simulink model "astolfi_278334"  (R2024b)
settings: Solver=ode113  StartTime=0.0  StopTime=60  RelTol=1e-10
values from neighbouring files (symbols this model uses):
  Ic = Iz + 2*Izz + 2*Mk*L*L    (= 7.5230625)    [Astolfi_278334.m]    (also in astolfi_278334.m)
  Ixx = (1/2)*Mk*Rk*Rk    (= 0.0140625)    [Astolfi_278334.m]    (also in astolfi_278334.m)
  k1 = 1    [Astolfi_278334.m]    (also in astolfi_278334.m)
  k2 = 10    [Astolfi_278334.m]    (also in astolfi_278334.m)
  Kd = 10    [Astolfi_278334.m]    (also in astolfi_278334.m)
  L = 0.3    [Astolfi_278334.m]    (also in astolfi_278334.m)
  Mc = Mp + 2*Mk    (= 107)    [Astolfi_278334.m]    (also in astolfi_278334.m)
  q0 = [1; 1;   pi;    0;    0]    [Astolfi_278334.m]    (also in astolfi_278334.m = [0; 0;   0;    0;    0])
  Rk = 0.075    [Astolfi_278334.m]    (also in astolfi_278334.m)
  thetad0 = 0    [Astolfi_278334.m]    (also in astolfi_278334.m)
  vd = wd*Rd    (= 1.0471975512)    [Astolfi_278334.m]    (also in astolfi_278334.m)
  wd = pi/6    (= 0.523598775598)    [Astolfi_278334.m]    (also in astolfi_278334.m)
  xd0 = 5    [Astolfi_278334.m]    (also in astolfi_278334.m)
  yd0 = -3    [Astolfi_278334.m]    (also in astolfi_278334.m)
settings Model: Creator=radek  LastModifiedBy=radek

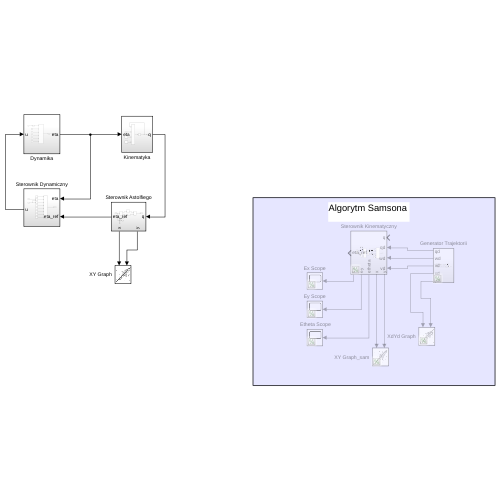
[thumbnail: Simulink's stored preview of the top-level diagram]
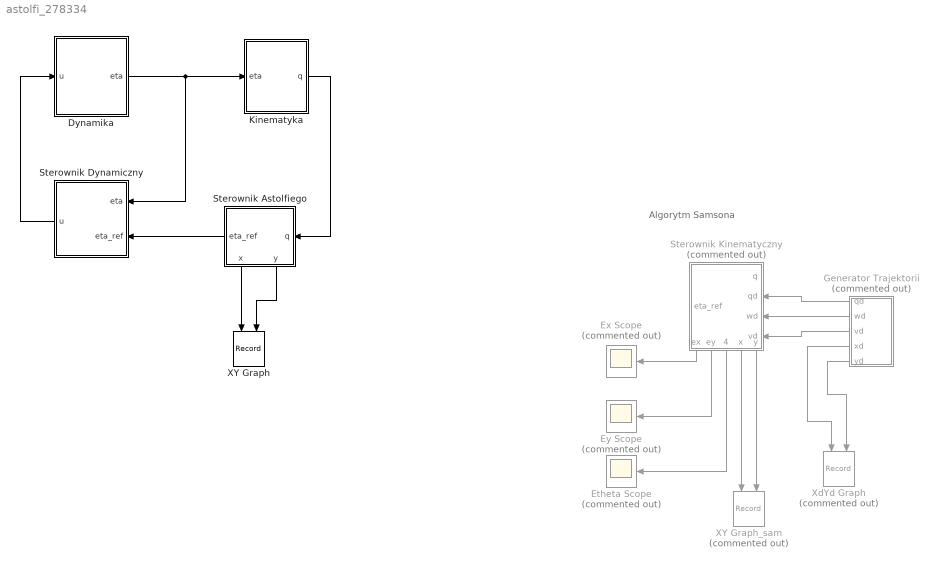
== system astolfi_278334 ==
  note: Algorytm Samsona
  " Etheta Scope" : Scope  Commented=on
  Dynamika : Subsystem
  Ex Scope : Scope  Commented=on
  Ey Scope : Scope  Commented=on
  Generator Trajektorii : Subsystem  Commented=on
  Kinematyka : Subsystem
  Sterownik Astolfiego : Subsystem
      settings: PortSchema="{\"entries\":[{\"content\":{\"sides\":[{\"content\":{\"connectorIds\":[\"In1\"]},\"type\":\"ConnectorPlacement.EquallySpacedRectSide\",\"uuid\":\"f5e69acf-f3ff-4fdf-98d6-c8734f1034ce\"},{\"content\":{\"connectorIds\":[\"Out1\"],\"side\":\"RIGHT\"},\"type\":\"ConnectorPlacement.EquallySpacedRectSide\",\"uuid\":\"aebf7805-5044-4096-9d39-e64456f3e00a\"},{\"content\":{\"side\":\"TOP\"},\"type\":\"ConnectorPlacement.EquallySpacedRectSide\",\"uuid\":\"74c1e2cd-73e2-4d01-a630-37efeb3275a2\"},{\"content\":{\"connectorIds\":[\"Out2\",\"Out3\"],\"side\":\"BOTTOM\"},\"type\":\"ConnectorPlacement.EquallySpacedRectSide\",\"uuid\":\"5cf9958d-65eb-4d7e-96d9-423271126dc6\"}]},\"type\":\"ConnectorPlacement.EquallySpacedConnector\",\"uuid\":\"6917b8e7-ecbe-45a3-8115-cac047f2c7ac\"}],\"packageUris\":[\"http://schema.mathworks.com/mf0/Connector/R2020b\"],\"version\":\"1.0\"}"
  Sterownik Dynamiczny : Subsystem
  Sterownik Kinematyczny : Subsystem  Commented=on
      settings: PortSchema="{\"entries\":[{\"content\":{\"sides\":[{\"content\":{\"connectorIds\":[\"In1\",\"In2\",\"In3\",\"In4\"]},\"type\":\"ConnectorPlacement.EquallySpacedRectSide\",\"uuid\":\"5192a1cc-ed77-4e56-a122-cfee3012277d\"},{\"content\":{\"connectorIds\":[\"Out1\"],\"side\":\"RIGHT\"},\"type\":\"ConnectorPlacement.EquallySpacedRectSide\",\"uuid\":\"40a037b4-09b0-4e17-a01c-e9007902fa24\"},{\"content\":{\"side\":\"TOP\"},\"type\":\"ConnectorPlacement.EquallySpacedRectSide\",\"uuid\":\"cd491b5b-2c4b-4e8a-9ff0-8dca4b136ad7\"},{\"content\":{\"connectorIds\":[\"Out2\",\"Out3\",\"Out4\",\"Out5\",\"Out6\"],\"side\":\"BOTTOM\"},\"type\":\"ConnectorPlacement.EquallySpacedRectSide\",\"uuid\":\"bb7d56d9-1ae6-4c8e-b63d-595b22e12c82\"}]},\"type\":\"ConnectorPlacement.EquallySpacedConnector\",\"uuid\":\"47c22155-c6cc-44ec-a96c-4ab3b3072b69\"}],\"packageUris\":[\"http://schema.mathworks.com/mf0/Connector/R2020b\"],\"version\":\"1.0\"}"
  XY Graph : Record  FileSettingsInternal="{\"entries\":[{\"content\":{\"excelSettings\":{\"content\":{},\"type\":\"Streamout.ExcelSettings\"}},\"type\":\"Streamout.FileSettingStorage\",\"uuid\":\"\"}],\"packageUris\":[\"http:\\/\\/schema.mathworks.com\\/mf0\\/streamout_blocks\\/R2020a\"],\"version\":\"1.0\"}"  Layout=[1 1]  SignalsInternal="{\"entries\":[{\"content\":{\"signals\":[{\"content\":{\"blockPath\":[],\"dimensions\":[1,1],\"domain\":\"\",\"lineColor\":\"#0072bd\",\"plots\":[ 1 ],\"port\":1,\"sid\":[\"\"],\"signalID\":1,\"signalName\":\"Sterownik Astolfiego:3\"},\"type\":\"RecordBlkView.Signal\",\"uuid\":\"\"},{\"content\":{\"blockPath\":[],\"dimensions\":[1,1],\"domain\":\"\",\"lineColor\":\"#d95319\",\"plots\":[ 1 ],\"port\":2,\"sid\":[\"\"],\"signalID\":2,\"signalName\":\"Sterownik Astolfiego:2\"},\"type\":\"RecordBlkView.Signal\",\"uuid\":\"\"}]},\"type\":\"RecordBlkView.InputSignals\",\"uuid\":\"\"}],\"packageUris\":[\"http:\\/\\/schema.mathworks.com\\/mf0\\/streamout_blocks\\/R2020a\"],\"version\":\"1.0\"}"  VisualizationBindings="{\"xyplotplugin\":{\"info\":[{\"series\":[{\"bindingParametersList\":[{\"parameter\":\"X-Axis\",\"signalID\":1,\"signalName\":\"Sterownik Astolfiego:3\"},{\"parameter\":\"Y-Axis\",\"signalID\":2,\"signalName\":\"Sterownik Astolfiego:2\"}],\"seriesID\":0}],\"subplotID\":1}]}}"  CompatibilityTag=XY
  XY Graph_sam : Record  Commented=on  FileSettingsInternal="{\"entries\":[{\"content\":{\"excelSettings\":{\"content\":{},\"type\":\"Streamout.ExcelSettings\"}},\"type\":\"Streamout.FileSettingStorage\",\"uuid\":\"\"}],\"packageUris\":[\"http:\\/\\/schema.mathworks.com\\/mf0\\/streamout_blocks\\/R2020a\"],\"version\":\"1.0\"}"  Layout=[1 1]  SignalsInternal="{\"entries\":[{\"content\":{\"signals\":[{\"content\":{\"blockPath\":[],\"dimensions\":[1],\"domain\":\"\",\"lineColor\":\"#0072bd\",\"plots\":[ 1 ],\"port\":1,\"signalID\":1,\"signalName\":\"Sterownik Kinematyczny:3\"},\"type\":\"RecordBlkView.Signal\",\"uuid\":\"\"},{\"content\":{\"blockPath\":[],\"dimensions\":[1],\"domain\":\"\",\"lineColor\":\"#d95319\",\"plots\":[ 1 ],\"port\":2,\"signalID\":2,\"signalName\":\"Sterownik Kinematyczny:2\"},\"type\":\"RecordBlkView.Signal\",\"uuid\":\"\"}]},\"type\":\"RecordBlkView.InputSignals\",\"uuid\":\"\"}],\"packageUris\":[\"http:\\/\\/schema.mathworks.com\\/mf0\\/streamout_blocks\\/R2020a\"],\"version\":\"1.0\"}"  VisualizationBindings="{\"xyplotplugin\":{\"info\":[{\"series\":[{\"bindingParametersList\":[{\"parameter\":\"X-Axis\",\"signalID\":1,\"signalName\":\"Sterownik Kinematyczny:3\"},{\"parameter\":\"Y-Axis\",\"signalID\":2,\"signalName\":\"Sterownik Kinematyczny:2\"}],\"seriesID\":0}],\"subplotID\":1}]}}"  CompatibilityTag=XY
  XdYd Graph : Record  Commented=on  FileSettingsInternal="{\"entries\":[{\"content\":{\"excelSettings\":{\"content\":{},\"type\":\"Streamout.ExcelSettings\"}},\"type\":\"Streamout.FileSettingStorage\",\"uuid\":\"\"}],\"packageUris\":[\"http:\\/\\/schema.mathworks.com\\/mf0\\/streamout_blocks\\/R2020a\"],\"version\":\"1.0\"}"  Layout=[1 1]  SignalsInternal="{\"entries\":[{\"content\":{\"signals\":[{\"content\":{\"blockPath\":[],\"dimensions\":[1],\"domain\":\"\",\"lineColor\":\"#a2142f\",\"plots\":[ 1 ],\"port\":1,\"signalID\":1,\"signalName\":\"Generator Trajektorii:4\"},\"type\":\"RecordBlkView.Signal\",\"uuid\":\"\"},{\"content\":{\"blockPath\":[],\"dimensions\":[1],\"domain\":\"\",\"lineColor\":\"#139fff\",\"plots\":[ 1 ],\"port\":2,\"signalID\":2,\"signalName\":\"Generator Trajektorii:5\"},\"type\":\"RecordBlkView.Signal\",\"uuid\":\"\"}]},\"type\":\"RecordBlkView.InputSignals\",\"uuid\":\"\"}],\"packageUris\":[\"http:\\/\\/schema.mathworks.com\\/mf0\\/streamout_blocks\\/R2020a\"],\"version\":\"1.0\"}"  VisualizationBindings="{\"xyplotplugin\":{\"info\":[{\"series\":[{\"bindingParametersList\":[{\"parameter\":\"X-Axis\",\"signalID\":1,\"signalName\":\"Generator Trajektorii:4\"},{\"parameter\":\"Y-Axis\",\"signalID\":2,\"signalName\":\"Generator Trajektorii:5\"}],\"seriesID\":0}],\"subplotID\":1}]}}"  CompatibilityTag=XY
  wires:
  Dynamika/1(eta) -> Sterownik Dynamiczny/1(eta), Kinematyka/1(eta)
  Sterownik Dynamiczny/1(u) -> Dynamika/1(u)
  Generator Trajektorii/1(qd) -> Sterownik Kinematyczny/2(qd)
  Generator Trajektorii/2(wd) -> Sterownik Kinematyczny/3(wd)
  Generator Trajektorii/3(vd) -> Sterownik Kinematyczny/4(vd)
  Sterownik Kinematyczny/3(x) -> XY Graph_sam/1
  Sterownik Kinematyczny/2(y) -> XY Graph_sam/2
  Generator Trajektorii/4(xd) -> XdYd Graph/1
  Generator Trajektorii/5(yd) -> XdYd Graph/2
  Sterownik Kinematyczny/6(ex) -> Ex Scope/1
  Sterownik Kinematyczny/5(ey) -> Ey Scope/1
  Sterownik Kinematyczny/4(etheta) -> " Etheta Scope"/1
  Sterownik Astolfiego/1(eta_ref) -> Sterownik Dynamiczny/2(eta_ref)
  Kinematyka/1(q) -> Sterownik Astolfiego/1(q)
  Sterownik Astolfiego/3(x) -> XY Graph/1
  Sterownik Astolfiego/2(y) -> XY Graph/2

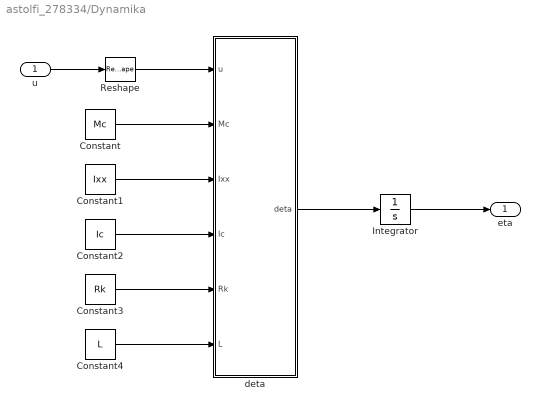
== system astolfi_278334/Dynamika ==
  u : Inport
  Constant : Constant  Value=Mc
  Constant1 : Constant  Value=Ixx
  Constant2 : Constant  Value=Ic
  Constant3 : Constant  Value=Rk
  Constant4 : Constant  Value=L
  Integrator : Integrator
  Reshape : Reshape  OutputDimensionality=Customize  OutputDimensions=[2,1]
  deta : MATLAB Function  TreatAsAtomicUnit=on
  eta : Outport
  wires:
  u/1 -> Reshape/1
  Constant1/1 -> deta/3(Ixx)
  Constant3/1 -> deta/5(Rk)
  Constant2/1 -> deta/4(Ic)
  Constant/1 -> deta/2(Mc)
  Constant4/1 -> deta/6(L)
  Integrator/1 -> eta/1
  deta/1(deta) -> Integrator/1
  Reshape/1 -> deta/1(u)

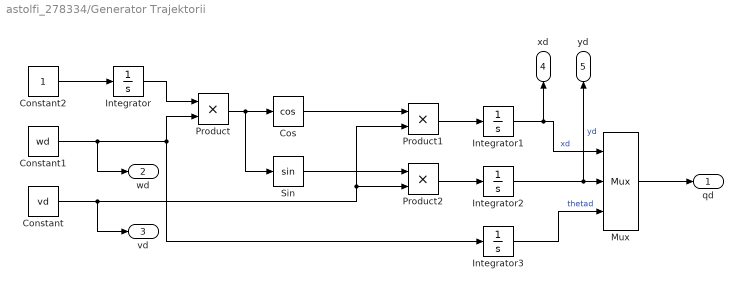
== system astolfi_278334/Generator Trajektorii ==
  Constant : Constant  Value=vd
  Constant1 : Constant  Value=wd
  Constant2 : Constant
  Cos : Trigonometry  Operator=cos
  Integrator : Integrator
  Integrator1 : Integrator  InitialCondition=xd0
  Integrator2 : Integrator  InitialCondition=yd0
  Integrator3 : Integrator  InitialCondition=thetad0
  Mux : Mux  Inputs=3
  Product : Product
  Product1 : Product
  Product2 : Product
  Sin : Trigonometry
  qd : Outport
  wd : Outport  Port=2
  vd : Outport  Port=3
  xd : Outport  Port=4
  yd : Outport  Port=5
  wires:
  Sin/1 -> Product2/1
  Constant2/1 -> Integrator/1
  Product2/1 -> Integrator2/1
  Product/1 -> Sin/1, Cos/1
  Cos/1 -> Product1/1
  Product1/1 -> Integrator1/1
  Integrator1/1 -> xd/1, Mux/1  "xd"
  Integrator/1 -> Product/1
  Constant1/1 -> wd/1, Product/2, Integrator3/1
  Mux/1 -> qd/1
  Integrator2/1 -> yd/1, Mux/2  "yd"
  Constant/1 -> vd/1, Product2/2, Product1/2
  Integrator3/1 -> Mux/3  "thetad"

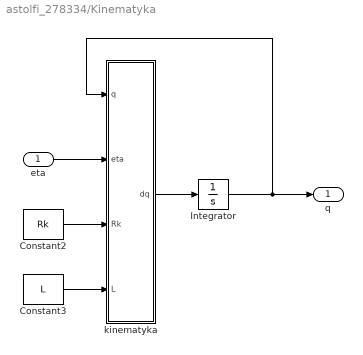
== system astolfi_278334/Kinematyka ==
  eta : Inport
  Constant2 : Constant  Value=Rk
  Constant3 : Constant  Value=L
  Integrator : Integrator  InitialCondition=q0
  kinematyka : MATLAB Function  TreatAsAtomicUnit=on
  q : Outport
  wires:
  Integrator/1 -> q/1, kinematyka/1(q)
  Constant3/1 -> kinematyka/4(L)
  eta/1 -> kinematyka/2(eta)
  Constant2/1 -> kinematyka/3(Rk)
  kinematyka/1(dq) -> Integrator/1

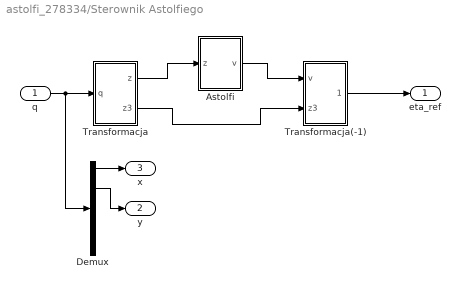
== system astolfi_278334/Sterownik Astolfiego ==
  q : Inport
  Astolfi : Subsystem
  Demux : Demux  Outputs=5
  Transformacja : Subsystem
  Transformacja(-1) : Subsystem
  eta_ref : Outport
  y : Outport  Port=2
  x : Outport  Port=3
  wires:
  q/1 -> Demux/1, Transformacja/1(q)
  Transformacja/1(z) -> Astolfi/1(z)
  Astolfi/1(v) -> Transformacja(-1)/1(v)
  Transformacja(-1)/1(eta_ref) -> eta_ref/1
  Transformacja/2(z3) -> Transformacja(-1)/2(z3)
  Demux/1 -> x/1
  Demux/2 -> y/1

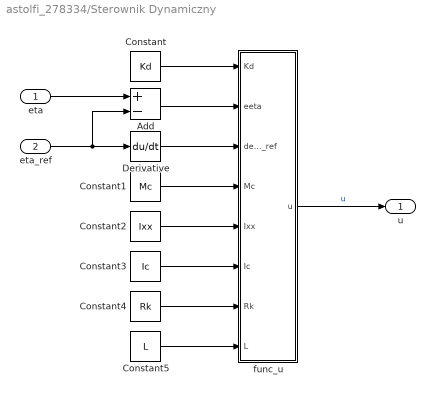
== system astolfi_278334/Sterownik Dynamiczny ==
  eta : Inport
  eta_ref : Inport  Port=2
  Add : Sum  Inputs=+-
  Constant : Constant  Value=Kd
  Constant1 : Constant  Value=Mc
  Constant2 : Constant  Value=Ixx
  Constant3 : Constant  Value=Ic
  Constant4 : Constant  Value=Rk
  Constant5 : Constant  Value=L
  Derivative : Derivative
  func_u : MATLAB Function  TreatAsAtomicUnit=on
  u : Outport
  wires:
  Constant1/1 -> func_u/4(Mc)
  eta/1 -> Add/1
  Constant3/1 -> func_u/6(Ic)
  Add/1 -> func_u/2(eeta)
  Derivative/1 -> func_u/3(deta_ref)
  Constant/1 -> func_u/1(Kd)
  Constant2/1 -> func_u/5(Ixx)
  func_u/1(u) -> u/1  "u"
  Constant4/1 -> func_u/7(Rk)
  eta_ref/1 -> Add/2, Derivative/1
  Constant5/1 -> func_u/8(L)

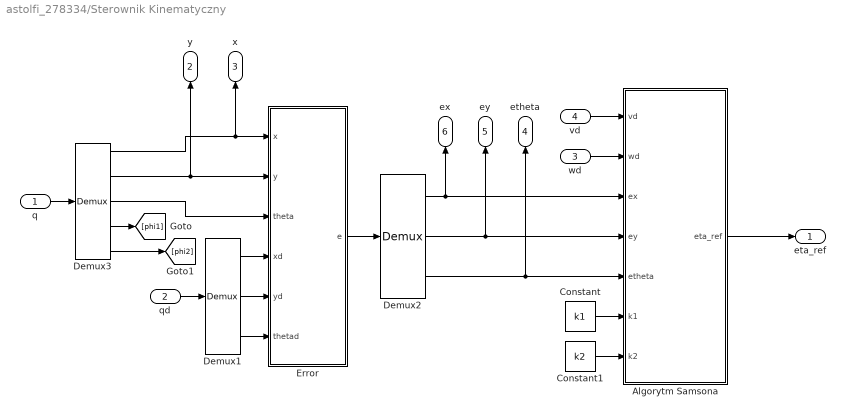
== system astolfi_278334/Sterownik Kinematyczny ==
  q : Inport
  qd : Inport  Port=2
  wd : Inport  Port=3
  vd : Inport  Port=4
  Algorytm Samsona : MATLAB Function  TreatAsAtomicUnit=on
  Constant : Constant  Value=k1
  Constant1 : Constant  Value=k2
  Demux1 : Demux  Outputs=3
      settings: DisplayOption=none
  Demux2 : Demux  Outputs=3
      settings: DisplayOption=none
  Demux3 : Demux  Outputs=5
      settings: DisplayOption=none
  Error : MATLAB Function  TreatAsAtomicUnit=on
  eta_ref : Outport
  y : Outport  Port=2
  x : Outport  Port=3
  etheta : Outport  Port=4
  ey : Outport  Port=5
  ex : Outport  Port=6
  wires:
  Demux1/1 -> Error/4(xd)
  Demux1/3 -> Error/6(thetad)
  Demux2/2 -> ey/1, Algorytm Samsona/4(ey)
  Algorytm Samsona/1(eta_ref) -> eta_ref/1
  Error/1(e) -> Demux2/1
  Demux2/3 -> etheta/1, Algorytm Samsona/5(etheta)
  Demux1/2 -> Error/5(yd)
  Demux2/1 -> ex/1, Algorytm Samsona/3(ex)
  Constant1/1 -> Algorytm Samsona/7(k2)
  Constant/1 -> Algorytm Samsona/6(k1)
  wd/1 -> Algorytm Samsona/2(wd)
  vd/1 -> Algorytm Samsona/1(vd)
  q/1 -> Demux3/1
  Demux3/3 -> Error/3(theta)
  Demux3/2 -> y/1, Error/2(y)
  qd/1 -> Demux1/1
  Demux3/1 -> x/1, Error/1(x)
  Demux3/4 -> [phi1]
  Demux3/5 -> [phi2]

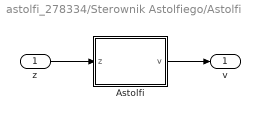
== system astolfi_278334/Sterownik Astolfiego/Astolfi ==
  z : Inport
  " Astolfi" : MATLAB Function  TreatAsAtomicUnit=on
  v : Outport
  wires:
  z/1 -> " Astolfi"/1(z)
  " Astolfi"/1(v) -> v/1

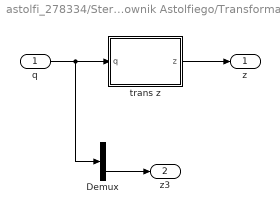
== system astolfi_278334/Sterownik Astolfiego/Transformacja ==
  q : Inport
  Demux : Demux  Outputs=3
  trans z : MATLAB Function  TreatAsAtomicUnit=on
  z : Outport
  z3 : Outport  Port=2
  wires:
  q/1 -> trans z/1(q), Demux/1
  Demux/3 -> z3/1
  trans z/1(z) -> z/1

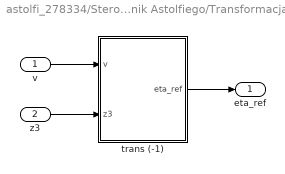
== system astolfi_278334/Sterownik Astolfiego/Transformacja(-1) ==
  v : Inport
  z3 : Inport  Port=2
  trans (-1) : MATLAB Function  TreatAsAtomicUnit=on
  eta_ref : Outport
  wires:
  trans (-1)/1(eta_ref) -> eta_ref/1
  v/1 -> trans (-1)/1(v)
  z3/1 -> trans (-1)/2(z3)

== matlab function astolfi_278334/Sterownik Kinematyczny/Error ==
  data: x input; e output; y input; theta input; xd input; yd input; thetad input
function e = e(x, y, theta, xd, yd, thetad)

    e_vec = [x - xd; y - yd; theta - thetad];
    ROT = [cos(thetad), sin(theta), 0; -sin(theta), cos(theta), 0; 0, 0, 1];

    e = ROT * e_vec;
    
end

== matlab function astolfi_278334/Kinematyka/kinematyka ==
  data: q input; dq output; eta input; Rk input; L input
function dq = dq(q, eta, Rk, L)
    theta = q(3);

    G2 = [cos(theta), 0;
          sin(theta), 0;
          0, 1;
          1/Rk, L/Rk;
          1/Rk, -L/Rk];

    dq = G2 * eta;
end

== matlab function astolfi_278334/Sterownik Kinematyczny/Algorytm Samsona ==
  data: eta_ref output; vd input; wd input; ex input; ey input; etheta input; k1 input; k2 input
function eta_ref = samson(vd, wd, ex, ey, etheta, k1, k2)

    if abs(etheta) > 0.000001
        setet = sin(etheta)/etheta;
    else
        setet = 1;
    end

    v = vd*cos(etheta) - k1*ex;
    w = wd - vd*ey*setet - k2*etheta; 
    eta_ref = [v; w];

end

== matlab function astolfi_278334/Dynamika/deta ==
  data: u input; Mc input; deta output; Ixx input; Ic input; Rk input; L input
function deta = deta(u, Mc, Ixx, Ic, Rk, L)

    M_star = [Mc + 2*Ixx/(Rk*Rk),      0; 
                0,        Ic + 2*Ixx*L*L/(Rk*Rk)];

    B_star = [1/Rk, 1/Rk; 
             L/Rk, -L/Rk];
    
    deta = M_star\B_star * u; % replaced inv(M)*B

end

== matlab function astolfi_278334/Sterownik Dynamiczny/func_u ==
  data: Kd input; u output; eeta input; deta_ref input; Mc input; Ixx input; Ic input; Rk input; L input
function u = u(Kd, eeta, deta_ref, Mc, Ixx, Ic, Rk, L)

    M_star = [Mc + 2*Ixx/(Rk*Rk), 0; 0, Ic + 2*Ixx*L*L/(Rk*Rk)];
    B_star = [1/Rk, 1/Rk; L/Rk, -L/Rk];

    u = inv(B_star)*M_star*(deta_ref - Kd*eeta);

end

== matlab function astolfi_278334/Sterownik Astolfiego/Transformacja/trans z ==
  data: q input; z output
function z = trans(q)

x = q(1);
y = q(2);
theta = q(3);

z1 = theta;
z2 = -x*cos(theta) - y*sin(theta);
z3 = -x*sin(theta) + y*cos(theta);

z = [z1;
     z2;
     z3];

end

== matlab function astolfi_278334/Sterownik Astolfiego/Transformacja(-1)/trans (-1) ==
  data: v input; eta_ref output; z3 input
function eta_ref = reverseTrans(v, z3)

v1 = v(1);
v2 = v(2);

omega_ref = v1;
v_ref = -v1*z3 - v2;

eta_ref = [omega_ref;
           v_ref];

end

== matlab function astolfi_278334/Sterownik Astolfiego/Astolfi/ Astolfi ==
  data: z input; v output
function v = astolfi(z)

% ---------MODYFIKOWALNE----------

k  =   1; % k > 0
p2 = -10; % p2 < -k
p3 =  20; % k * (p2 + p3) > 0

% --------------------------------

z1 = z(1);
z2 = z(2);
z3 = z(3);

if (abs(z) < 0.000001)

    v1 = -k * z1;
    v2 = -p2*z2 + p3*(z3/z1);
  
else

    v1 = 0;
    v2 = 0;
   
end

v = [v1;
     v2];

end
